simulink model "psbwindgen"  (Simulink 6.0)
settings: Solver=ode23tb  StartTime=0.0  StopTime=3  RelTol=1e-4
PreLoadFcn:
  | load psbwindgen_data
InitFcn:
  | powericon('psbinitsys',bdroot);
values from neighbouring files (symbols this model uses):
  psbwindgen_char = [0 0 0 0 0 0 0 0 0 0 0.02551 0.02551 ... (243 elements, 9x27)]    [power_windgen_init.mat]
undefined symbols (not defined in the file or in its folder): gcbh, powericon
libraries: powerlib2 x50, powerlib_extras x5
(part 1 of 2)
settings Model: Creator=gagnonr  LastModifiedBy=batserve  ExtModeAutoUpdateStatusClock=off  ProdHWDeviceType=Specified
settings DataIOCC: LimitDataPoints=off  LoadInitialState=on  SaveFinalState=on  SaveOutput=off  SignalLoggingName=sigsOut
settings OptimizationCC: BlockReduction=off  BooleanDataType=off
settings DebuggingCC: CheckExecutionContextPreStartOutputMsg=on  CheckExecutionContextRuntimeOutputMsg=on  SolverPrmCheckMsg=none
settings HardwareCC: ProdBitPerShort=32  ProdBitPerInt=16  ProdHWDeviceType=Specified  TargetUnknown=on

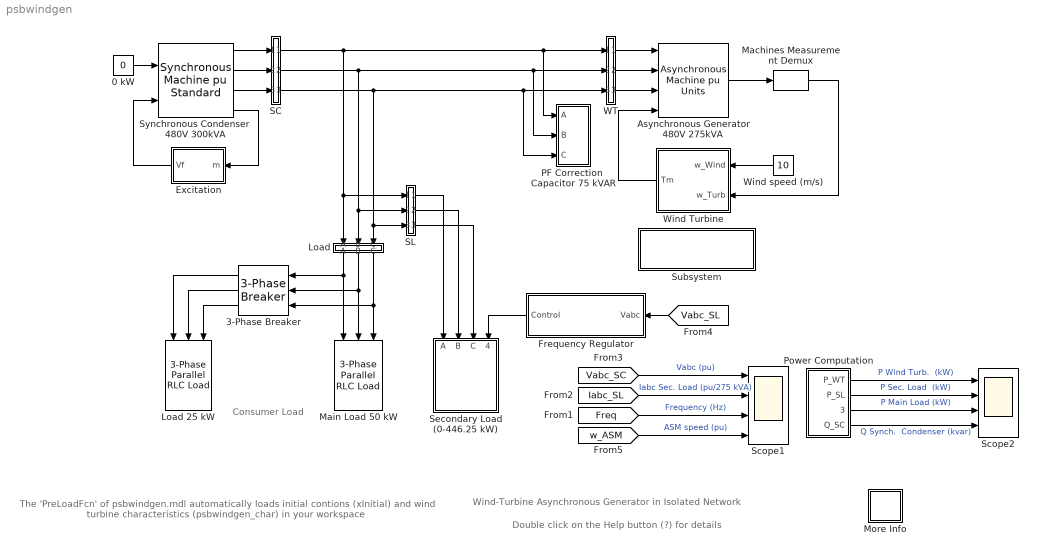
== system psbwindgen ==
  note: Double click on the Help button (?) for details
  note: Wind-Turbine Asynchronous Generator in Isolated Network
  note: The 'PreLoadFcn' of psbwindgen.mdl automatically
      | loads initial contions (xInitial)
      | and wind turbine characteristics (psbwindgen_char)
      | in your workspace
  note: Consumer Load
  0 kW : Constant  Value=0
  3-Phase Breaker : powerlib2/Elements/3-Phase Breaker  Orientation=left  init_states=open  sa=on  sb=on  sc=on  sw_times=[0.2]  Ts=0  comext=off  Ron=0.001  Rp=1e6  Cp=inf  mesure=None
  Asynchronous Generator 480V 275kVA : powerlib2/Machines/Asynchronous Machine pu Units  Tag=PoWeRsYsTeMbLoCk  rotType=Squirrel-cage  ctrl=Rotor  x1=[ 275e3, 480, 60 ]  x2=[ 0.016,0.06]  x3=[ 0.015,0.06]  x4=3.5  x5=[ 2,0,2 ]  x6=[-8.89496e-048 0 0.280896 0.280896 0.280896 -89.7425 150.258 30.2575]  PSBOutputType=1110  iounits=0  LoadFlowParameters=0
  Excitation : Subsystem  Orientation=left
  Frequency Regulator : Subsystem  Orientation=left  mask(Frequency regulator){Vpp_nom=460, Freq=60, gains_regulator=[150 70], Phref=1}
      mask prompts: Vpp_nom "Phase to phase voltage (Vrms):"; Freq "Reference frequency (Hz):"; gains_regulator "Regulator gains  [Kp Kd]:"; Phref "Reference phase (rd):"
      mask help:
      | Frequency regulator
      |
      | Input : phase to ground voltages
      |
      | Output : 24 logical signals for the control of the dump load
      mask init:
      | Vbase=Vpp_nom/sqrt(3);
      | Kp=gains_regulator(1);
      | Kd=gains_regulator(2);
  Load : Subsystem  Tag=PoWeRsYsTeMmEaSuReMeNt  Orientation=down  AncestorBlock=powerlib2/Measurements/Three-Phase V-I Measurement  LoadFcn=powericon('psbloadfunction',gcbh,'3-Phase VI Measurement','');  InitFcn=powericon('checksum',bdroot)  mask(3-Phase VI Measurement){VChoice=phase-to-ground, ualv=on, labelV=Vabc_Load, Vpu=on, Vbase=480, IChoice=yes, ualc=on, labelC=Iabc_Load, Ppu=on, Pbase=275e3, OutputType=Magnitude, PhasorSimulation=off, PSBequivalent=0, PSBOutputType=11100}
      mask prompts: VChoice "Voltage measurement"; ualv "Use a label"; labelV "Signal label  (use a From block to collect signal)"; Vpu "Voltage  in pu"; Vbase "Base voltage (Vrms phase-phase) :"; IChoice "Current measurement"; ualc "Use a label"; labelC "Signal label  (use a From block to collect signal)"; Ppu "Currents in pu"; Pbase "Base power ( VA 3 phase)"; OutputType "Output signal :"; PhasorSimulation "Phasor simulation"; PSBequivalent "Equivalent circuit"
      mask help:
      | This block is used to measure three-phase voltages and currents in a circuit. When connected in series with a three-phase element, it return the three phase-to-ground voltages and line currents.
      |
      | The block can output the voltages and currents in per unit values or in volts and amperes. Check the appropriate boxes if you want to output the voltages and currents  in pu
      mask init:
      | powericon('psbcallbacks',gcb,'Three-phase measurements',4);
      | if  Vpu
      |     xKv=1/(Vbase/sqrt(3)*sqrt(2));
      | else
      |     xKv=1;
      | end
      | if  Ppu
      |     xKi=1/(Pbase/Vbase/sqrt(3)*sqrt(2));
      | else
      |     xKi=1;
      | end
      | switch OutputType
      | case 1
      |     OutputSelection  = [1:6];
      |     PhasorModeV = [1:3];
      |     NormalModeV = [7:9];
      |     PhasorModeI = [4:6];
      |     NormalModeI = [10:12];
      |     Kv = xKv;
      |     Ki = xKi;
      | case 2
      |     OutputSelection = [7,13,8,14,9,15,10,16,11,17,12,18];
      |     PhasorModeV = [1:6];
      |     NormalModeV = [13:15];
      |     PhasorModeI = [7:12];
      |     NormalModeI = [16:18];
      |     Kv = xKv;
      |     Ki = xKi;
      | case 3
      |     OutputSelection = [13,19,14,20,15,21,16,22,17,23,18,24];
      |     PhasorModeV = [1:6];
      |     NormalModeV = [13:15];
      |     PhasorModeI = [7:12];
      |     NormalModeI = [16:18];
      |     Kv = [xKv 1 xKv 1 xKv 1];
      |     Ki = [xKi 1 xKi 1 xKi 1];
      | case 4
      |     OutputSelection  = [19:24];
      |     PhasorModeV = [1:3];
      |     NormalModeV = [7:9];
      |     PhasorModeI = [4:6];
      |     NormalModeI = [10:12];
      |     Kv = xKv;
      |     Ki = xKi;
      | end
      | if PhasorSimulation
      |     SelectionModeV = PhasorModeV;
      |     SelectionModeI = PhasorModeI;
      | else
      |     SelectionModeV = NormalModeV;
      |     SelectionModeI = NormalModeI;
      |     Kv = xKv;
      |     Ki = xKi;
      | end
      settings: CopyFcn=powericon('psbloadfunction',gcbh,'3-Phase VI Measurement','VerifyPhasor');  CloseFcn=%3phaseVImeasurement
      mask Help: web(psbhelp)
      mask StyleString: popup(no|phase-to-ground|phase-to-phase),checkbox,edit,checkbox,edit,popup(no|yes),checkbox,edit,checkbox,edit,popup(Complex|Real-Imag|Magnitude-Angle|Magnitude),checkbox,edit,edit
      mask CallbackString: powericon('psbcallbacks',gcb,'Three-phase measurements',2);|powericon('psbcallbacks',gcb,'Three-phase measurements',2);||powericon('psbcallbacks',gcb,'Three-phase measurements',2);||powericon('psbcallbacks',gcb,'Three-phase measurements',2);|powericon('psbcallbacks',gcb,'Three-phase measurements',2);||powericon('psbcallbacks',gcb,'Three-phase measurements',4);|||||
  Load 25 kW : powerlib2/Elements/3-Phase Parallel RLC Load  Orientation=down  Vpp=480  fn=60  P3=25e3  QL3=0  QC3=0
  Machines Measurement Demux : powerlib2/Machines/Machines Measurement Demux  machType=Asynchronous  ssm1=on  ssm2=on  ssm3=on  ssm4=on  ssm5=on  ssm6=on  sm1=off  sm2=off  sm3=off  sm4=off  sm5=off  sm6=off  sm7=off  sm8=on  sm9=off  sm10=off  sm11=off  sm115=off  sm12=off  sm13=off  sm14=off  asm1=off  asm2=off  asm3=off  asm4=off  asm5=off  asm6=off  asm7=off  asm8=off  asm9=on  asm10=off  asm11=off  pmsm1=on  pmsm2=on  pmsm3=on  pmsm4=on  pmsm5=on  pmsm6=on  lastType=1
  Main Load 50 kW : powerlib2/Elements/3-Phase Parallel RLC Load  Orientation=down  Vpp=480  fn=60  P3=50e3  QL3=0  QC3=0
  More Info : Subsystem
      mask Display: disp('?')
  PF Correction  Capacitor 75 kVAR : Subsystem
  Power Computation : Subsystem
  SC : Subsystem  Tag=PoWeRsYsTeMmEaSuReMeNt  AncestorBlock=powerlib2/Measurements/Three-Phase V-I Measurement  LoadFcn=powericon('psbloadfunction',gcbh,'3-Phase VI Measurement','');  InitFcn=powericon('checksum',bdroot)  mask(3-Phase VI Measurement){VChoice=phase-to-ground, ualv=on, labelV=Vabc_SC, Vpu=on, Vbase=480, IChoice=yes, ualc=on, labelC=Iabc_SC, Ppu=on, Pbase=300e3, OutputType=Magnitude, PhasorSimulation=off, PSBequivalent=0, PSBOutputType=11100}
      mask prompts: VChoice "Voltage measurement"; ualv "Use a label"; labelV "Signal label  (use a From block to collect signal)"; Vpu "Voltage  in pu"; Vbase "Base voltage (Vrms phase-phase) :"; IChoice "Current measurement"; ualc "Use a label"; labelC "Signal label  (use a From block to collect signal)"; Ppu "Currents in pu"; Pbase "Base power ( VA 3 phase)"; OutputType "Output signal :"; PhasorSimulation "Phasor simulation"; PSBequivalent "Equivalent circuit"
      mask help:
      | This block is used to measure three-phase voltages and currents in a circuit. When connected in series with a three-phase element, it return the three phase-to-ground voltages and line currents.
      |
      | The block can output the voltages and currents in per unit values or in volts and amperes. Check the appropriate boxes if you want to output the voltages and currents  in pu
      mask init: same as psbwindgen/Load
      settings: CopyFcn=powericon('psbloadfunction',gcbh,'3-Phase VI Measurement','VerifyPhasor');  CloseFcn=%3phaseVImeasurement
      mask Help: web(psbhelp)
      mask StyleString: popup(no|phase-to-ground|phase-to-phase),checkbox,edit,checkbox,edit,popup(no|yes),checkbox,edit,checkbox,edit,popup(Complex|Real-Imag|Magnitude-Angle|Magnitude),checkbox,edit,edit
      mask CallbackString: powericon('psbcallbacks',gcb,'Three-phase measurements',2);|powericon('psbcallbacks',gcb,'Three-phase measurements',2);||powericon('psbcallbacks',gcb,'Three-phase measurements',2);||powericon('psbcallbacks',gcb,'Three-phase measurements',2);|powericon('psbcallbacks',gcb,'Three-phase measurements',2);||powericon('psbcallbacks',gcb,'Three-phase measurements',4);|||||
  SL : Subsystem  Tag=PoWeRsYsTeMmEaSuReMeNt  AncestorBlock=powerlib2/Measurements/Three-Phase V-I Measurement  LoadFcn=powericon('psbloadfunction',gcbh,'3-Phase VI Measurement','');  InitFcn=powericon('checksum',bdroot)  mask(3-Phase VI Measurement){VChoice=phase-to-ground, ualv=on, labelV=Vabc_SL, Vpu=on, Vbase=480, IChoice=yes, ualc=on, labelC=Iabc_SL, Ppu=on, Pbase=275e3, OutputType=Magnitude, PhasorSimulation=off, PSBequivalent=0, PSBOutputType=11100}
      mask prompts: VChoice "Voltage measurement"; ualv "Use a label"; labelV "Signal label  (use a From block to collect signal)"; Vpu "Voltage  in pu"; Vbase "Base voltage (Vrms phase-phase) :"; IChoice "Current measurement"; ualc "Use a label"; labelC "Signal label  (use a From block to collect signal)"; Ppu "Currents in pu"; Pbase "Base power ( VA 3 phase)"; OutputType "Output signal :"; PhasorSimulation "Phasor simulation"; PSBequivalent "Equivalent circuit"
      mask help:
      | This block is used to measure three-phase voltages and currents in a circuit. When connected in series with a three-phase element, it return the three phase-to-ground voltages and line currents.
      |
      | The block can output the voltages and currents in per unit values or in volts and amperes. Check the appropriate boxes if you want to output the voltages and currents  in pu
      mask init: same as psbwindgen/Load
      settings: CopyFcn=powericon('psbloadfunction',gcbh,'3-Phase VI Measurement','VerifyPhasor');  CloseFcn=%3phaseVImeasurement
      mask Help: web(psbhelp)
      mask StyleString: popup(no|phase-to-ground|phase-to-phase),checkbox,edit,checkbox,edit,popup(no|yes),checkbox,edit,checkbox,edit,popup(Complex|Real-Imag|Magnitude-Angle|Magnitude),checkbox,edit,edit
      mask CallbackString: powericon('psbcallbacks',gcb,'Three-phase measurements',2);|powericon('psbcallbacks',gcb,'Three-phase measurements',2);||powericon('psbcallbacks',gcb,'Three-phase measurements',2);||powericon('psbcallbacks',gcb,'Three-phase measurements',2);|powericon('psbcallbacks',gcb,'Three-phase measurements',2);||powericon('psbcallbacks',gcb,'Three-phase measurements',4);|||||
  Scope1 : Scope  NumInputPorts=4
      settings: TimeRange=3  YMin=-1.5~-0.75~59.5~1.005  YMax=1.5~0.75~60.5~1.015  SaveName=Vabc
  Scope2 : Scope  NumInputPorts=4
      settings: TimeRange=3  YMin=180~100~40~0  YMax=250~200~80~35  SaveName=Power  DataFormat=Array
  Secondary Load (0-446.25 kW) : Subsystem  Orientation=down  mask(8-step Variable Load){Vphase_phase_lissage=480, Freq=60, P_lissage_min=1.75e3, Pin_3phase=50e3}
      mask prompts: Vphase_phase_lissage "Nominal L-L voltage (Vrms):"; Freq "Nominal frequency (Hz):"; P_lissage_min "Power per step Pstep (W):"; Pin_3phase "Initial power  (W) :"
      mask help:
      | This block implements a variable, three-phase resistive load. The load variation uses an eight-bit binary progression so that the load power can be varied by steps from 0 to 255*Pstep.
      |
      | The eight three-phase resistors are connected in series with ideal switches simulating forced-commutated power electronic switches.
      |
      | The Pulses input is a vector containing the eight bits (0/1) controlling the eight three-phase switches. First value is the less significant bit.
      mask init:
      | Ron_switch=1e-6;
      | Rs_snubber=inf;
      | Cs_snubber=0;
      | n_niveaux=8;
      | Pmax=((2^n_niveaux)-1)*P_lissage_min;
      | Pin_normalise=min([(Pin_3phase/Pmax)*((2^n_niveaux)-1) ((2^n_niveaux)-1)]);
      | discret1=pow2(0:-1:-(n_niveaux-1))*Pin_normalise;
      | discret2=floor(discret1);
      | Status=rem(discret2,2);
  Subsystem : Subsystem
      settings: OpenFcn=open('psbwindgen_turb.fig')
      mask Display: disp('Double click to display\nTurbine characteristics')
  Synchronous Condenser  480V 300kVA : powerlib2/Machines/Synchronous Machine pu Standard  Tag=PoWeRsYsTeMbLoCk  rotorType=Salient-pole  x1=[ 300e3 480 60 ]  x2b=[ 3.23, 0.21, 0.15, 2.79, 1.03, 0.37, 0.09 ]  x2=[ 3.23, 0.21, 0.15, 2.79, 0.37, 0.09]  dAxisT=Open-circuit  qAxisT=Open-circuit  x3a="[ 1.7  0.008  0.004]"  x3b=[ 1.7, 0.008, 0.213, 0.004 ]  x3c="[  1.7 0.008 0.051266  ]"  x3d=[ 8.0, 0.03, 0.3371, 0.0295 ]  x3="[ 0.08  0.019  0.004 ]"  x3e=[ 1.3201, 0.023, 1.0, 0.07 ]  x3f="[  0.08  0.019 0.051266  ]"  x3g=[ 1.3201, 0.0231, 0.3371, 0.0295 ]  x4=0.017  x5=[ 1, 0, 2 ]  x6=[0 -89.2146 0.827 0.827 0.827 -86.4 153.6 33.6 2.71455]  x7=off  x8=[0.6404,0.7127,0.8441,0.9214,0.9956,1.082,1.19,1.316,1.457;0.7,0.7698,0.8872,0.9466,0.9969,1.046,1.1,1.151,1.201]  PSBOutputType=1110  iounits=0.5  LoadFlowParameters=[2 0 0 0 0]
  WT : Subsystem  Tag=PoWeRsYsTeMmEaSuReMeNt  AncestorBlock=powerlib2/Measurements/Three-Phase V-I Measurement  LoadFcn=powericon('psbloadfunction',gcbh,'3-Phase VI Measurement','');  InitFcn=powericon('checksum',bdroot)  mask(3-Phase VI Measurement){VChoice=phase-to-ground, ualv=on, labelV=Vabc_WT, Vpu=on, Vbase=480, IChoice=yes, ualc=on, labelC=Iabc_WT, Ppu=on, Pbase=275e3, OutputType=Magnitude, PhasorSimulation=off, PSBequivalent=0, PSBOutputType=11100}
      mask prompts: VChoice "Voltage measurement"; ualv "Use a label"; labelV "Signal label  (use a From block to collect signal)"; Vpu "Voltage  in pu"; Vbase "Base voltage (Vrms phase-phase) :"; IChoice "Current measurement"; ualc "Use a label"; labelC "Signal label  (use a From block to collect signal)"; Ppu "Currents in pu"; Pbase "Base power ( VA 3 phase)"; OutputType "Output signal :"; PhasorSimulation "Phasor simulation"; PSBequivalent "Equivalent circuit"
      mask help:
      | This block is used to measure three-phase voltages and currents in a circuit. When connected in series with a three-phase element, it return the three phase-to-ground voltages and line currents.
      |
      | The block can output the voltages and currents in per unit values or in volts and amperes. Check the appropriate boxes if you want to output the voltages and currents  in pu
      mask init: same as psbwindgen/Load
      settings: CopyFcn=powericon('psbloadfunction',gcbh,'3-Phase VI Measurement','VerifyPhasor');  CloseFcn=%3phaseVImeasurement
      mask Help: web(psbhelp)
      mask StyleString: popup(no|phase-to-ground|phase-to-phase),checkbox,edit,checkbox,edit,popup(no|yes),checkbox,edit,checkbox,edit,popup(Complex|Real-Imag|Magnitude-Angle|Magnitude),checkbox,edit,edit
      mask CallbackString: powericon('psbcallbacks',gcb,'Three-phase measurements',2);|powericon('psbcallbacks',gcb,'Three-phase measurements',2);||powericon('psbcallbacks',gcb,'Three-phase measurements',2);||powericon('psbcallbacks',gcb,'Three-phase measurements',2);|powericon('psbcallbacks',gcb,'Three-phase measurements',2);||powericon('psbcallbacks',gcb,'Three-phase measurements',4);|||||
  Wind Turbine : Subsystem  Orientation=left
  Wind speed (m/s) : Constant  Orientation=left  Value=10
  wires:
  Load/3("C ") -> Main Load 50 kW/3, 3-Phase Breaker/3
  0 kW/1 -> Synchronous Condenser  480V 300kVA/1
  Synchronous Condenser  480V 300kVA/4 -> Excitation/1(m)
  Excitation/1(Vf) -> Synchronous Condenser  480V 300kVA/2
  [Freq] -> Scope1/3  "Frequency (Hz)"
  [Vabc_SC] -> Scope1/1  "Vabc (pu)"
  Load/1("A ") -> Main Load 50 kW/1, 3-Phase Breaker/1
  Load/2("B ") -> Main Load 50 kW/2, 3-Phase Breaker/2
  WT/1("A ") -> Asynchronous Generator 480V 275kVA/1
  WT/2("B ") -> Asynchronous Generator 480V 275kVA/2
  WT/3("C ") -> Asynchronous Generator 480V 275kVA/3
  Synchronous Condenser  480V 300kVA/1 -> SC/1(A)
  Synchronous Condenser  480V 300kVA/2 -> SC/2(B)
  Synchronous Condenser  480V 300kVA/3 -> SC/3(C)
  SC/1("A ") -> PF Correction  Capacitor 75 kVAR/1(A), WT/1(A), SL/1(A), Load/1(A)
  SC/2("B ") -> PF Correction  Capacitor 75 kVAR/2(B), WT/2(B), SL/2(B), Load/2(B)
  SC/3("C ") -> PF Correction  Capacitor 75 kVAR/3(C), WT/3(C), SL/3(C), Load/3(C)
  [Iabc_SL] -> Scope1/2  "Iabc Sec. Load (pu/275 kVA)"
  3-Phase Breaker/1 -> Load 25 kW/1
  3-Phase Breaker/2 -> Load 25 kW/2
  3-Phase Breaker/3 -> Load 25 kW/3
  Asynchronous Generator 480V 275kVA/1 -> Machines Measurement Demux/1
  Machines Measurement Demux/1 -> Wind Turbine/2(w_Turb)
  Wind speed (m/s)/1 -> Wind Turbine/1(w_Wind)
  [Vabc_SL] -> Frequency Regulator/1(Vabc)
  Power Computation/1(P_WT) -> Scope2/1  "P Wind Turb.  (kW)"
  Power Computation/2(P_SL) -> Scope2/2  "P Sec. Load  (kW)"
  Power Computation/3(P_Load) -> Scope2/3  "P Main Load (kW)"
  Power Computation/4(Q_SC) -> Scope2/4  "Q Synch.  Condenser (kvar)"
  Wind Turbine/1(Tm) -> Asynchronous Generator 480V 275kVA/4
  SL/1("A ") -> Secondary Load (0-446.25 kW)/1(A)
  SL/2("B ") -> Secondary Load (0-446.25 kW)/2(B)
  SL/3("C ") -> Secondary Load (0-446.25 kW)/3(C)
  Frequency Regulator/1(Control) -> Secondary Load (0-446.25 kW)/4(Control)
  [w_ASM] -> Scope1/4  "ASM speed (pu)"

== system psbwindgen/Excitation ==
  m : Inport  Orientation=left  Port=1  LatchInput=off
  Constant3 : Constant  Orientation=left
  Demux : Demux  Orientation=left  Outputs=2
  Excitation System : powerlib2/Machines/Excitation System  Orientation=left  tr=20e-3  reg=[ 300, 0.001 ]  exc=[ 1, 0 ]  tgr=[ 0, 0 ]  damp=[ 0.001, 0.1 ]  sat=[ 0, 0 ]  lim=[ -11.5, 11.5, 0 ]  v0=[1,2.71455]
  Gain : Gain  Gain=60  SaturateOnIntegerOverflow=on
  Ground : Ground  Orientation=left
  Machines Measurement Demux : powerlib2/Machines/Machines Measurement Demux  Orientation=left  machType=Synchronous  ssm1=on  ssm2=on  ssm3=on  ssm4=on  ssm5=on  ssm6=on  sm1=off  sm2=off  sm3=off  sm4=off  sm5=off  sm6=on  sm7=off  sm8=on  sm9=off  sm10=off  sm11=off  sm115=off  sm12=off  sm13=off  sm14=off  asm1=on  asm2=on  asm3=on  asm4=on  asm5=on  asm6=on  asm7=on  asm8=on  asm9=on  asm10=on  asm11=on  pmsm1=on  pmsm2=on  pmsm3=on  pmsm4=on  pmsm5=on  pmsm6=on  lastType=1
  Vf : Outport  Orientation=left
  tag scope: Freq=global
  wires:
  Machines Measurement Demux/1 -> Demux/1
  Demux/1 -> Excitation System/3
  Demux/2 -> Excitation System/2
  Constant3/1 -> Excitation System/1
  Ground/1 -> Excitation System/4
  Machines Measurement Demux/2 -> Gain/1
  m/1 -> Machines Measurement Demux/1
  Excitation System/1 -> Vf/1
  Gain/1 -> [Freq]

== system psbwindgen/Frequency Regulator ==
  Vabc : Inport  Port=1  LatchInput=off
  3-phase PLL : powerlib_extras/Control  Blocks/3-phase PLL  Par_Init=[0 Freq]  ParK=[60 1400]
  Frequency : Constant  Value=Freq
  Integrator : Integrator  LimitOutput=on  UpperSaturationLimit=6  LowerSaturationLimit=-1
  PD : Subsystem
  Phref : Constant  Value=Phref
  Pulses Decoder : Subsystem  mask(Pulses Decoder){n=8}
      mask prompts: n "Number of bits to decode:"
      mask help:
      | Decode the scalar input 'Code' into a vector output 'Pulses' based on  the specified number of bits to decode.
      | (Element 1 of vector output = least significant bit)
  Sampling system : Subsystem
  Sum : Sum  Inputs=|+-  SaturateOnIntegerOverflow=on  InputSameDT=on
  Sum1 : Sum  Inputs=|+-  SaturateOnIntegerOverflow=on  InputSameDT=on
  Terminator : Terminator
  Terminator1 : Terminator
  Control : Outport
  wires:
  Vabc/1 -> 3-phase PLL/1
  3-phase PLL/3 -> Terminator1/1
  3-phase PLL/2 -> Terminator/1
  3-phase PLL/1 -> Sum/1
  Sampling system/1(Pulses_ABC0_7) -> Control/1
  Phref/1 -> Sum1/2
  Sum1/1 -> PD/1(In)
  Integrator/1 -> Sum1/1
  Frequency/1 -> Sum/2
  PD/1(Out) -> Pulses Decoder/1(Code)
  Sum/1 -> Integrator/1
  Pulses Decoder/1(Pulses) -> Sampling system/1(BITA0_7)

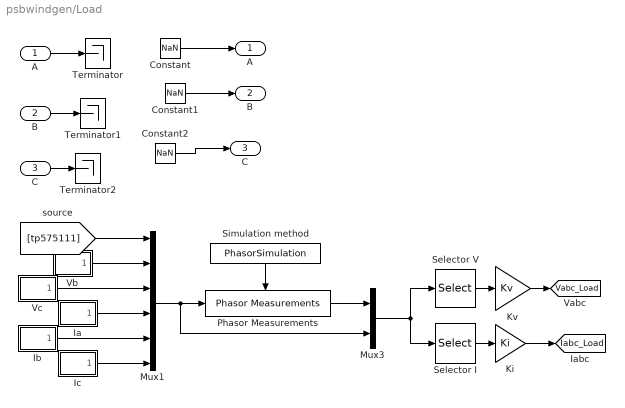
== system psbwindgen/Load ==
  A : Inport  Port=1  LatchInput=off
  B : Inport  Port=2  LatchInput=off
  C : Inport  Port=3  LatchInput=off
  Constant : Constant  Value=NaN
  Constant1 : Constant  Value=NaN
  Constant2 : Constant  Value=NaN
  Ia : Subsystem  AncestorBlock=powerlib2/Measurements/Three-Phase V-I Measurement/Ia
  Ib : Subsystem  AncestorBlock=powerlib2/Measurements/Three-Phase V-I Measurement/Ib
  Ic : Subsystem  AncestorBlock=powerlib2/Measurements/Three-Phase V-I Measurement/Ic
  Ki : Gain  Gain=Ki  SaturateOnIntegerOverflow=on
  Kv : Gain  Gain=Kv  SaturateOnIntegerOverflow=on
  Mux1 : Mux  Inputs=6
  Mux3 : Mux  Inputs=2
  Phasor Measurements : powerlib2/Measurements/Three-Phase V-I Measurement/Phasor Measurements  TreatAsAtomicUnit=on  SimViewingDevice=off  DataTypeOverride=UseLocalSettings  MinMaxOverflowLogging=UseLocalSettings
      settings: Permissions=ReadWrite  RTWFcnNameOpts=Auto  RTWFileNameOpts=Auto
  Selector I : Selector  Elements=SelectionModeI  InputPortWidth=length(OutputSelection)+6
  Selector V : Selector  Elements=SelectionModeV  InputPortWidth=length(OutputSelection)+6
  Simulation method : Constant  Orientation=down  Value=PhasorSimulation
  Terminator : Terminator
  Terminator1 : Terminator
  Terminator2 : Terminator
  Vb : Subsystem  AncestorBlock=powerlib2/Measurements/Three-Phase V-I Measurement/Vb
  Vc : Subsystem  AncestorBlock=powerlib2/Measurements/Three-Phase V-I Measurement/Vc
  "A " : Outport
  "B " : Outport  Port=2
  "C " : Outport  Port=3
  tag scope: Iabc_Load=global, Vabc_Load=global
  wires:
  Ic/1(Out1) -> Mux1/6
  Ib/1(Out1) -> Mux1/5
  Ia/1(Out1) -> Mux1/4
  Vc/1(Out1) -> Mux1/3
  Vb/1(Out1) -> Mux1/2
  [tp575111] -> Mux1/1
  Mux1/1 -> Phasor Measurements/1, Mux3/2
  Simulation method/1 -> Phasor Measurements/Enable
  Phasor Measurements/1 -> Mux3/1
  Mux3/1 -> Selector V/1, Selector I/1
  Selector I/1 -> Ki/1
  Selector V/1 -> Kv/1
  Ki/1 -> [Iabc_Load]
  Kv/1 -> [Vabc_Load]
  Constant2/1 -> "C "/1
  Constant1/1 -> "B "/1
  Constant/1 -> "A "/1
  C/1 -> Terminator2/1
  B/1 -> Terminator1/1
  A/1 -> Terminator/1

== system psbwindgen/More Info ==
  note: [1] R. Gagnon, B. Saulnier, G. Sybille, P. Giroux; "Modeling of a Generic High-Penetration No-Storage Wind-Diesel System Using Matlab/Power System Blockset"
      | 2002 Global Windpower Conference, April 2002, Paris, France
      | [2] B. Saulnier, A.O. Barry, B. Dube, R. Reid; "Design and Development of a Regulation and Control System for the High-Penetration No-Storage Wind/Diesel
      | Scheme" European Community Wind Energy Conference 88, 6-10 june 1988, Herning, Denmark
      | [3] L. Mott (NPS), B. Saulnier (IREQ) " Commercial Wind-Diesel Project, St. Paul Island, Alaska" 14th Prime Power Diesel Inter-Utility Conference,
      | May 28-June 2, Winnipeg, Manitoba, Canada
  note: References
  note: For the demo, the wind speed (10m/s) is such that the wind turbine produces enough power to supply the load. The diesel-generator (not simulated) is stopped
      | and the the synchronous machine operates as a synchronous condenser with its mechanical power input (Pm) set at zero.
      | The demo illustrates the dynamic performance of the frequency regulation system when an additional 25 kW customer load is switched on.
      |
      | Start simulation and observe voltages, currents, powers, asynchronous machine speed and system frequency on the two scopes.
      | Initial conditions (xInitial vector) have been automatically loaded in your workspace so that simulation starts in steady state.
      |
      | As the asynchronous machine operates in generator mode, its speed is slightly above the synchronous speed (1.011 pu).
      | According to turbine characteristics, for a 10m/s wind speed, the turbine output power is 0.75 pu (206 kW). Because of the asynchronous machine losses,
      | the wind turbine produces 200 kW. As the main load is 50 kW, the secondary load absorbs 150 kW to maintain a constant 60 Hz frequency.
      | At t=0.2 s, the additional load of 25 kW is switched on. The frequency  momentarily drops to 59.8 Hz and the frequency regulator reacts to reduce the power
      | absorbed by the secondary load in order to bring the frequency back to 60 Hz. Voltage stays at 1 pu and no flicker is observed.
  note: R. Reid, B. Saulnier, R. Gagnon; Hydro-Quebec (IREQ)
  note: A generic model of the High-Penetration, No Storage, Wind-Diesel (HPNSWD) system is presented in this demo [1].
      | This technology was developed by Hydro-Quebec to reduce the cost of supplying electricity in remote northern communities[2].
      | The optimal wind penetration (installed wind capacity/peak electrical demand) for this system depends on the site delivery cost of fuel
      | and available wind resource. The first commercial application of HPNSWD technology was commissioned in 1999 by Northern Power Systems (Vermont,USA)
      | on St. Paul Island, Alaska [3]. The HPNSWD system presented in this demo uses a 480 V, 300 kVA synchronous machine, a wind turbine driving
      | a 480 V, 275 kVA induction generator, a 50 kW customer load and a variable secondary load (0 to 446.25 kW).
      |
      | At low wind speeds both the induction generator and the diesel-driven synchronous generator are required to feed the load.
      | When the wind power exceeds the load demand, it is possible to shut down the diesel-generator. In this all-wind mode, the synchronous machine
      | is used as a synchronous condenser and its excitation system controls the grid voltage at its nominal value.
      | A secondary load bank is used to regulate the system frequency by absorbing the wind power exceeding consumer demand.
      |
      | The Wind Turbine block uses a 2-D Lookup Table to compute the turbine torque output (Tm) as a function of wind speed (w_Wind) and turbine speed (w_Turb).
      | When you opened this demo, the Pm(w_Wind, w_Turb) characteristics was automatically loaded in your workspace (psbwindgen_char array).
      | To display the turbine characteristics, double click on the block located below the Wind Turbine block.
      |
      | The Secondary Load block consists of eight sets of three-phase resistors connected in series with GTO thyristor switches.
      | The nominal power of each set follows a binary progression so that the load can be varied from 0 to 446.25 kW by steps of 1.75kW.
      | GTOs are simulated by ideal switches.
      |
      | The Frequency Regulator uses a standard three-phase Phase Locked Loop (PLL) system to measure the system frequency.
      | The measured frequency is compared to the reference frequency (60 Hz) to obtain the frequency error. This error is integrated to obtain the
      | phase error. The phase error is then used  by a Proportional-Differential (PD) controller to produce an output signal representing the required
      | secondary load power. This analog signal is converted to an 8-bit digital signal controlling switching of the eight three-phase secondary loads.
      | In order to minimize voltage disturbances, switching is performed at zero crossing of voltage.
  note: Wind-Turbine Asynchronous Generator in Isolated Network
  note: Circuit Description
  note: Demonstration

== system psbwindgen/PF Correction  Capacitor 75 kVAR ==
  A : Inport  Orientation=left  Port=1  LatchInput=off
  B : Inport  Orientation=left  Port=2  LatchInput=off
  C : Inport  Orientation=left  Port=3  LatchInput=off
  L connector : powerlib2/Connectors/L connector  Tag=PoWeRsYsTeMbLoCk
  L connector1 : powerlib2/Connectors/L connector  Tag=PoWeRsYsTeMbLoCk
  L connector2 : powerlib2/Connectors/L connector  Tag=PoWeRsYsTeMbLoCk
  Series RLC Load : powerlib2/Elements/Series RLC Load  Tag=PoWeRsYsTeMbLoCk  a=480  b=60  c=0  d=0  e=25e3  mesure=None  PSBOutputType=1
  Series RLC Load2 : powerlib2/Elements/Series RLC Load  Tag=PoWeRsYsTeMbLoCk  a=480  b=60  c=0  d=0  e=25e3  mesure=None  PSBOutputType=1
  Series RLC Load3 : powerlib2/Elements/Series RLC Load  Tag=PoWeRsYsTeMbLoCk  a=480  b=60  c=0  d=0  e=25e3  mesure=None  PSBOutputType=1
  wires:
  C/1 -> L connector2/Enable
  B/1 -> L connector1/Enable
  A/1 -> L connector/Enable
  Series RLC Load2/1 -> L connector2/1, Series RLC Load/1
  Series RLC Load3/1 -> L connector1/1, Series RLC Load2/1
  Series RLC Load/1 -> L connector/1, Series RLC Load3/1

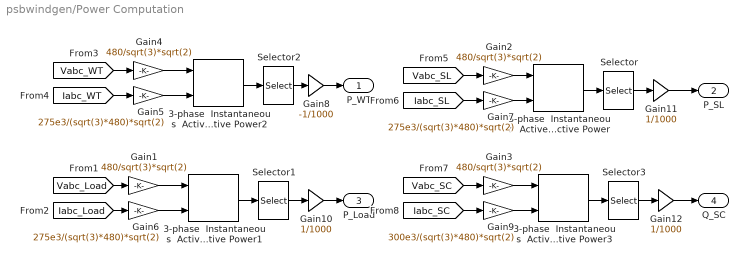
== system psbwindgen/Power Computation ==
  3-phase  Instantaneous  Active & Reactive Power{,1..3} (4 alike) : powerlib_extras/Measurements/3-phase  Instantaneous  Active & Reactive Power
  Gain{1..4} (4 alike) : Gain  Gain=480/sqrt(3)*sqrt(2)  SaturateOnIntegerOverflow=on
  Gain10 : Gain  Gain=1/1000  SaturateOnIntegerOverflow=on
  Gain11 : Gain  Gain=1/1000  SaturateOnIntegerOverflow=on
  Gain12 : Gain  Gain=1/1000  SaturateOnIntegerOverflow=on
  Gain5 : Gain  Gain=275e3/(sqrt(3)*480)*sqrt(2)  SaturateOnIntegerOverflow=on
  Gain6 : Gain  Gain=275e3/(sqrt(3)*480)*sqrt(2)  SaturateOnIntegerOverflow=on
  Gain7 : Gain  Gain=275e3/(sqrt(3)*480)*sqrt(2)  SaturateOnIntegerOverflow=on
  Gain8 : Gain  Gain=-1/1000  SaturateOnIntegerOverflow=on
  Gain9 : Gain  Gain=300e3/(sqrt(3)*480)*sqrt(2)  SaturateOnIntegerOverflow=on
  Selector : Selector  Elements=[1]  InputPortWidth=2
  Selector1 : Selector  Elements=[1]  InputPortWidth=2
  Selector2 : Selector  Elements=[1]  InputPortWidth=2
  Selector3 : Selector  Elements=[2]  InputPortWidth=2
  P_WT : Outport
  P_SL : Outport  Port=2
  P_Load : Outport  Port=3
  Q_SC : Outport  Port=4
  wires:
  3-phase  Instantaneous  Active & Reactive Power/1 -> Selector/1
  Selector/1 -> Gain11/1
  3-phase  Instantaneous  Active & Reactive Power1/1 -> Selector1/1
  3-phase  Instantaneous  Active & Reactive Power2/1 -> Selector2/1
  [Vabc_WT] -> Gain4/1
  [Iabc_WT] -> Gain5/1
  3-phase  Instantaneous  Active & Reactive Power3/1 -> Selector3/1
  Gain4/1 -> 3-phase  Instantaneous  Active & Reactive Power2/1
  Gain5/1 -> 3-phase  Instantaneous  Active & Reactive Power2/2
  [Vabc_Load] -> Gain1/1
  [Iabc_Load] -> Gain6/1
  Gain1/1 -> 3-phase  Instantaneous  Active & Reactive Power1/1
  Gain6/1 -> 3-phase  Instantaneous  Active & Reactive Power1/2
  [Vabc_SL] -> Gain2/1
  [Iabc_SL] -> Gain7/1
  Gain2/1 -> 3-phase  Instantaneous  Active & Reactive Power/1
  Gain7/1 -> 3-phase  Instantaneous  Active & Reactive Power/2
  Selector1/1 -> Gain10/1
  Selector2/1 -> Gain8/1
  Gain8/1 -> P_WT/1
  Selector3/1 -> Gain12/1
  [Vabc_SC] -> Gain3/1
  [Iabc_SC] -> Gain9/1
  Gain3/1 -> 3-phase  Instantaneous  Active & Reactive Power3/1
  Gain9/1 -> 3-phase  Instantaneous  Active & Reactive Power3/2
  Gain10/1 -> P_Load/1
  Gain11/1 -> P_SL/1
  Gain12/1 -> Q_SC/1

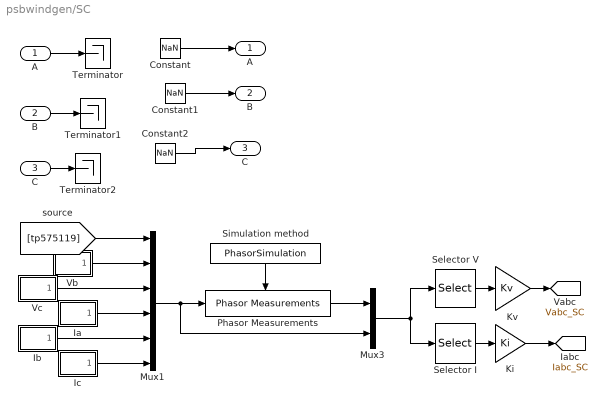
== system psbwindgen/SC ==
  A : Inport  Port=1  LatchInput=off
  B : Inport  Port=2  LatchInput=off
  C : Inport  Port=3  LatchInput=off
  Constant : Constant  Value=NaN
  Constant1 : Constant  Value=NaN
  Constant2 : Constant  Value=NaN
  Ia : Subsystem  AncestorBlock=powerlib2/Measurements/Three-Phase V-I Measurement/Ia
  Ib : Subsystem  AncestorBlock=powerlib2/Measurements/Three-Phase V-I Measurement/Ib
  Ic : Subsystem  AncestorBlock=powerlib2/Measurements/Three-Phase V-I Measurement/Ic
  Ki : Gain  Gain=Ki  SaturateOnIntegerOverflow=on
  Kv : Gain  Gain=Kv  SaturateOnIntegerOverflow=on
  Mux1 : Mux  Inputs=6
  Mux3 : Mux  Inputs=2
  Phasor Measurements : powerlib2/Measurements/Three-Phase V-I Measurement/Phasor Measurements  TreatAsAtomicUnit=on  SimViewingDevice=off  DataTypeOverride=UseLocalSettings  MinMaxOverflowLogging=UseLocalSettings
      settings: Permissions=ReadWrite  RTWFcnNameOpts=Auto  RTWFileNameOpts=Auto
  Selector I : Selector  Elements=SelectionModeI  InputPortWidth=length(OutputSelection)+6
  Selector V : Selector  Elements=SelectionModeV  InputPortWidth=length(OutputSelection)+6
  Simulation method : Constant  Orientation=down  Value=PhasorSimulation
  Terminator : Terminator
  Terminator1 : Terminator
  Terminator2 : Terminator
  Vb : Subsystem  AncestorBlock=powerlib2/Measurements/Three-Phase V-I Measurement/Vb
  Vc : Subsystem  AncestorBlock=powerlib2/Measurements/Three-Phase V-I Measurement/Vc
  "A " : Outport
  "B " : Outport  Port=2
  "C " : Outport  Port=3
  tag scope: Iabc_SC=global, Vabc_SC=global
  wires:
  A/1 -> Terminator/1
  B/1 -> Terminator1/1
  C/1 -> Terminator2/1
  Constant/1 -> "A "/1
  Constant1/1 -> "B "/1
  Constant2/1 -> "C "/1
  Kv/1 -> [Vabc_SC]
  Ki/1 -> [Iabc_SC]
  Selector V/1 -> Kv/1
  Selector I/1 -> Ki/1
  Mux3/1 -> Selector I/1, Selector V/1
  Phasor Measurements/1 -> Mux3/1
  Simulation method/1 -> Phasor Measurements/Enable
  Mux1/1 -> Mux3/2, Phasor Measurements/1
  [tp575119] -> Mux1/1
  Vb/1(Out1) -> Mux1/2
  Vc/1(Out1) -> Mux1/3
  Ia/1(Out1) -> Mux1/4
  Ib/1(Out1) -> Mux1/5
  Ic/1(Out1) -> Mux1/6

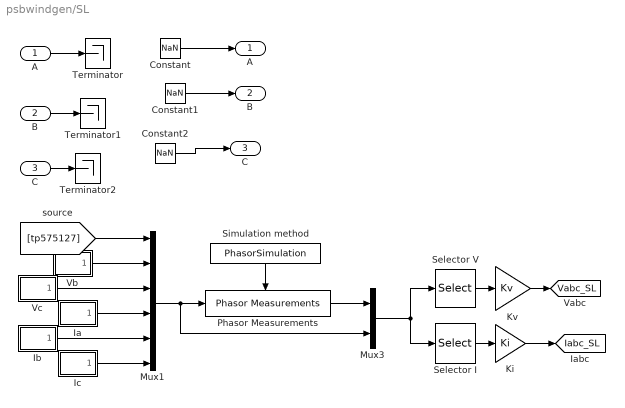
== system psbwindgen/SL ==
  A : Inport  Port=1  LatchInput=off
  B : Inport  Port=2  LatchInput=off
  C : Inport  Port=3  LatchInput=off
  Constant : Constant  Value=NaN
  Constant1 : Constant  Value=NaN
  Constant2 : Constant  Value=NaN
  Ia : Subsystem  AncestorBlock=powerlib2/Measurements/Three-Phase V-I Measurement/Ia
  Ib : Subsystem  AncestorBlock=powerlib2/Measurements/Three-Phase V-I Measurement/Ib
  Ic : Subsystem  AncestorBlock=powerlib2/Measurements/Three-Phase V-I Measurement/Ic
  Ki : Gain  Gain=Ki  SaturateOnIntegerOverflow=on
  Kv : Gain  Gain=Kv  SaturateOnIntegerOverflow=on
  Mux1 : Mux  Inputs=6
  Mux3 : Mux  Inputs=2
  Phasor Measurements : powerlib2/Measurements/Three-Phase V-I Measurement/Phasor Measurements  TreatAsAtomicUnit=on  SimViewingDevice=off  DataTypeOverride=UseLocalSettings  MinMaxOverflowLogging=UseLocalSettings
      settings: Permissions=ReadWrite  RTWFcnNameOpts=Auto  RTWFileNameOpts=Auto
  Selector I : Selector  Elements=SelectionModeI  InputPortWidth=length(OutputSelection)+6
  Selector V : Selector  Elements=SelectionModeV  InputPortWidth=length(OutputSelection)+6
  Simulation method : Constant  Orientation=down  Value=PhasorSimulation
  Terminator : Terminator
  Terminator1 : Terminator
  Terminator2 : Terminator
  Vb : Subsystem  AncestorBlock=powerlib2/Measurements/Three-Phase V-I Measurement/Vb
  Vc : Subsystem  AncestorBlock=powerlib2/Measurements/Three-Phase V-I Measurement/Vc
  "A " : Outport
  "B " : Outport  Port=2
  "C " : Outport  Port=3
  tag scope: Iabc_SL=global, Vabc_SL=global
  wires:
  A/1 -> Terminator/1
  B/1 -> Terminator1/1
  C/1 -> Terminator2/1
  Constant/1 -> "A "/1
  Constant1/1 -> "B "/1
  Constant2/1 -> "C "/1
  Kv/1 -> [Vabc_SL]
  Ki/1 -> [Iabc_SL]
  Selector V/1 -> Kv/1
  Selector I/1 -> Ki/1
  Mux3/1 -> Selector I/1, Selector V/1
  Phasor Measurements/1 -> Mux3/1
  Simulation method/1 -> Phasor Measurements/Enable
  Mux1/1 -> Mux3/2, Phasor Measurements/1
  [tp575127] -> Mux1/1
  Vb/1(Out1) -> Mux1/2
  Vc/1(Out1) -> Mux1/3
  Ia/1(Out1) -> Mux1/4
  Ib/1(Out1) -> Mux1/5
  Ic/1(Out1) -> Mux1/6

== system psbwindgen/Secondary Load (0-446.25 kW) ==
  A : Inport  Port=1  LatchInput=off
  B : Inport  Port=2  LatchInput=off
  C : Inport  Port=3  LatchInput=off
  Control : Inport  Port=4  LatchInput=off
  Demux : Demux  Outputs=8
  Resistive Loads : Subsystem
  Switches : Subsystem
  wires:
  Control/1 -> Demux/1
  Demux/8 -> Switches/11(P_ABC7)
  Demux/7 -> Switches/10(P_ABC6)
  Demux/6 -> Switches/9(P_ABC5)
  Demux/5 -> Switches/8(P_ABC4)
  Demux/4 -> Switches/7(P_ABC3)
  Demux/3 -> Switches/6(P_ABC2)
  Demux/2 -> Switches/5(P_ABC1)
  Demux/1 -> Switches/4(P_ABC0)
  C/1 -> Switches/3(C)
  B/1 -> Switches/2(B)
  A/1 -> Switches/1(A)
  Switches/24(C7) -> Resistive Loads/24(C7)
  Switches/23(B7) -> Resistive Loads/23(B7)
  Switches/22(A7) -> Resistive Loads/22(A7)
  Switches/21(C6) -> Resistive Loads/21(C6)
  Switches/20(B6) -> Resistive Loads/20(B6)
  Switches/19(A6) -> Resistive Loads/19(A6)
  Switches/18(C5) -> Resistive Loads/18(C5)
  Switches/17(B5) -> Resistive Loads/17(B5)
  Switches/16(A5) -> Resistive Loads/16(A5)
  Switches/15(C4) -> Resistive Loads/15(C4)
  Switches/14(B4) -> Resistive Loads/14(B4)
  Switches/13(A4) -> Resistive Loads/13(A4)
  Switches/12(C3) -> Resistive Loads/12(C3)
  Switches/11(B3) -> Resistive Loads/11(B3)
  Switches/10(A3) -> Resistive Loads/10(A3)
  Switches/9(C2) -> Resistive Loads/9(C2)
  Switches/8(B2) -> Resistive Loads/8(B2)
  Switches/7(A2) -> Resistive Loads/7(A2)
  Switches/6(C1) -> Resistive Loads/6(C1)
  Switches/5(B1) -> Resistive Loads/5(B1)
  Switches/4(A1) -> Resistive Loads/4(A1)
  Switches/3(C0) -> Resistive Loads/3(C0)
  Switches/2(B0) -> Resistive Loads/2(B0)
  Switches/1(A0) -> Resistive Loads/1(A0)

== system psbwindgen/Subsystem ==

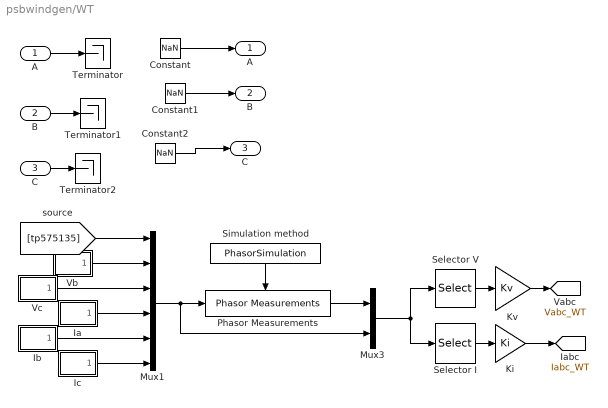
== system psbwindgen/WT ==
  A : Inport  Port=1  LatchInput=off
  B : Inport  Port=2  LatchInput=off
  C : Inport  Port=3  LatchInput=off
  Constant : Constant  Value=NaN
  Constant1 : Constant  Value=NaN
  Constant2 : Constant  Value=NaN
  Ia : Subsystem  AncestorBlock=powerlib2/Measurements/Three-Phase V-I Measurement/Ia
  Ib : Subsystem  AncestorBlock=powerlib2/Measurements/Three-Phase V-I Measurement/Ib
  Ic : Subsystem  AncestorBlock=powerlib2/Measurements/Three-Phase V-I Measurement/Ic
  Ki : Gain  Gain=Ki  SaturateOnIntegerOverflow=on
  Kv : Gain  Gain=Kv  SaturateOnIntegerOverflow=on
  Mux1 : Mux  Inputs=6
  Mux3 : Mux  Inputs=2
  Phasor Measurements : powerlib2/Measurements/Three-Phase V-I Measurement/Phasor Measurements  TreatAsAtomicUnit=on  SimViewingDevice=off  DataTypeOverride=UseLocalSettings  MinMaxOverflowLogging=UseLocalSettings
      settings: Permissions=ReadWrite  RTWFcnNameOpts=Auto  RTWFileNameOpts=Auto
  Selector I : Selector  Elements=SelectionModeI  InputPortWidth=length(OutputSelection)+6
  Selector V : Selector  Elements=SelectionModeV  InputPortWidth=length(OutputSelection)+6
  Simulation method : Constant  Orientation=down  Value=PhasorSimulation
  Terminator : Terminator
  Terminator1 : Terminator
  Terminator2 : Terminator
  Vb : Subsystem  AncestorBlock=powerlib2/Measurements/Three-Phase V-I Measurement/Vb
  Vc : Subsystem  AncestorBlock=powerlib2/Measurements/Three-Phase V-I Measurement/Vc
  "A " : Outport
  "B " : Outport  Port=2
  "C " : Outport  Port=3
  tag scope: Iabc_WT=global, Vabc_WT=global
  wires:
  Ic/1(Out1) -> Mux1/6
  Ib/1(Out1) -> Mux1/5
  Ia/1(Out1) -> Mux1/4
  Vc/1(Out1) -> Mux1/3
  Vb/1(Out1) -> Mux1/2
  [tp575135] -> Mux1/1
  Mux1/1 -> Phasor Measurements/1, Mux3/2
  Simulation method/1 -> Phasor Measurements/Enable
  Phasor Measurements/1 -> Mux3/1
  Mux3/1 -> Selector V/1, Selector I/1
  Selector I/1 -> Ki/1
  Selector V/1 -> Kv/1
  Ki/1 -> [Iabc_WT]
  Kv/1 -> [Vabc_WT]
  Constant2/1 -> "C "/1
  Constant1/1 -> "B "/1
  Constant/1 -> "A "/1
  C/1 -> Terminator2/1
  B/1 -> Terminator1/1
  A/1 -> Terminator/1

== system psbwindgen/Wind Turbine ==
  w_Wind : Inport  Port=1  LatchInput=off
  w_Turb : Inport  Port=2  LatchInput=off
  1800 rpm : Gain  Gain=1800  SaturateOnIntegerOverflow=on
  Constant3 : Constant  Value=1e-6
  Gain : Gain  Gain=-1  SaturateOnIntegerOverflow=on
  P(w_Wind,w_Turb) : Lookup2D  DialogController=Simulink.DDGSource  RowIndex=[0 5 6 7 8 9 10 11 12]  ColumnIndex=[0 571.55 685.8 800.15 914.4 1028.8 1143.1 1257.4 1371.7 1486 1600.3 1714.6 1828.9 1943.2 2057.5 2171.8 2286.1 2400.5 2514.7 2629.1 2743.3 2857.7 2971.9 3086.3 3200.5 3314.9 3429.2]  OutputValues=psbwindgen_char  SaturateOnIntegerOverflow=on  InputSameDT=on
  Product : Product  Inputs=*/  SaturateOnIntegerOverflow=on  InputSameDT=on
  Switch : Switch  Threshold=1e-6  SaturateOnIntegerOverflow=on  InputSameDT=on
  Tm : Outport
  tag scope: w_ASM=global
  wires:
  w_Turb/1 -> 1800 rpm/1, Switch/1, Switch/2, [w_ASM]
  Constant3/1 -> Switch/3
  w_Wind/1 -> P(w_Wind,w_Turb)/1
  P(w_Wind,w_Turb)/1 -> Product/1
  Switch/1 -> Product/2
  Product/1 -> Gain/1
  Gain/1 -> Tm/1
  1800 rpm/1 -> P(w_Wind,w_Turb)/2

== system psbwindgen/Frequency Regulator/PD ==
  In : Inport  Port=1  LatchInput=off
  "0, 255" : Saturate  UpperLimit=255  LowerLimit=0
  Gain I : Gain  Gain=Kd  SaturateOnIntegerOverflow=on
  Gain P : Gain  Gain=Kp  SaturateOnIntegerOverflow=on
  Sum : Sum  SaturateOnIntegerOverflow=on  InputSameDT=on
  Transfer Fcn : TransferFcn  Numerator=[1 0]  Denominator=[1e-3 1]
  Out : Outport
  wires:
  Transfer Fcn/1 -> Sum/2
  "0, 255"/1 -> Out/1
  Gain I/1 -> Transfer Fcn/1
  In/1 -> Gain P/1, Gain I/1
  Gain P/1 -> Sum/1
  Sum/1 -> "0, 255"/1

== system psbwindgen/Frequency Regulator/Pulses Decoder ==
  Code : Inport  Port=1  LatchInput=off
  Constant : Constant  Value=pow2(0:-1:-(n-1))
  Constant6 : Constant  Value=2
  Math Function : Math  Operator=rem  SaturateOnIntegerOverflow=on
  Product : Product  SaturateOnIntegerOverflow=on  InputSameDT=on
  Rounding Function : Rounding
  Pulses : Outport
  wires:
  Math Function/1 -> Pulses/1
  Rounding Function/1 -> Math Function/1
  Constant6/1 -> Math Function/2
  Product/1 -> Rounding Function/1
  Code/1 -> Product/1
  Constant/1 -> Product/2

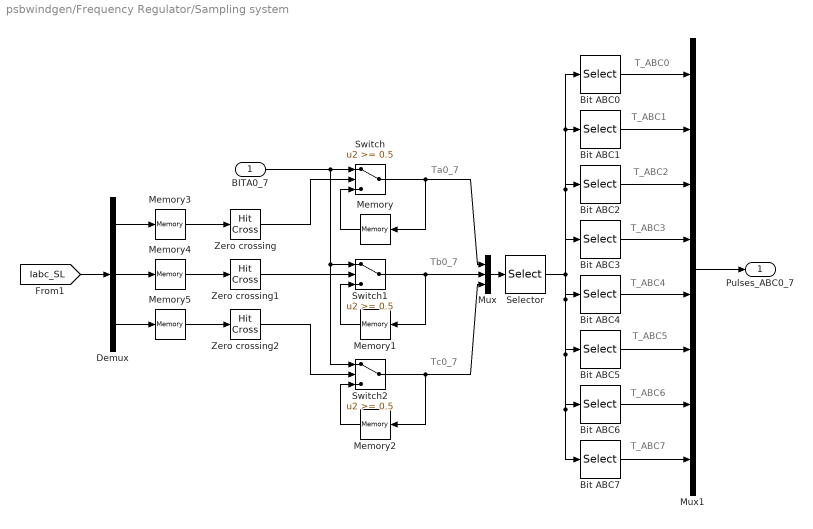
== system psbwindgen/Frequency Regulator/Sampling system ==
  note: T_ABC7
  note: T_ABC6
  note: T_ABC5
  note: T_ABC4
  note: T_ABC3
  note: T_ABC2
  note: T_ABC1
  note: T_ABC0
  note: Tc0_7
  note: Tb0_7
  note: Ta0_7
  BITA0_7 : Inport  Port=1  LatchInput=off
  " Bit ABC4" : Selector  Elements=[13 14 15]  InputPortWidth=24
  Bit ABC0 : Selector  Elements=[1 2 3]  InputPortWidth=24
  Bit ABC1 : Selector  Elements=[4 5 6]  InputPortWidth=24
  Bit ABC2 : Selector  Elements=[7 8 9]  InputPortWidth=24
  Bit ABC3 : Selector  Elements=[10 11 12]  InputPortWidth=24
  Bit ABC5 : Selector  Elements=[16 17 18]  InputPortWidth=24
  Bit ABC6 : Selector  Elements=[19 20 21]  InputPortWidth=24
  Bit ABC7 : Selector  Elements=[22 23 24]  InputPortWidth=24
  Demux : Demux  Outputs=3
  Memory : Memory  Orientation=left
  Memory1 : Memory  Orientation=left
  Memory2 : Memory  Orientation=left
  Memory3 : Memory
  Memory4 : Memory
  Memory5 : Memory
  Mux : Mux  Inputs=3
  Mux1 : Mux  Inputs=8
  Selector : Selector  Elements=[1 9 17 2 10 18 3 11 19 4 12 20 5 13 21 6 14 22 7 15 23 8 16 24]  InputPortWidth=24
  Switch : Switch  Threshold=0.5  SaturateOnIntegerOverflow=on  InputSameDT=on
  Switch1 : Switch  Threshold=0.5  SaturateOnIntegerOverflow=on  InputSameDT=on
  Switch2 : Switch  Threshold=0.5  SaturateOnIntegerOverflow=on  InputSameDT=on
  Zero crossing : HitCross
  Zero crossing1 : HitCross
  Zero crossing2 : HitCross
  Pulses_ABC0_7 : Outport
  wires:
  BITA0_7/1 -> Switch2/1, Switch1/1, Switch/1
  Memory5/1 -> Zero crossing2/1
  Memory4/1 -> Zero crossing1/1
  Memory3/1 -> Zero crossing/1
  Demux/3 -> Memory5/1
  Demux/2 -> Memory4/1
  Demux/1 -> Memory3/1
  Zero crossing2/1 -> Switch2/2
  Zero crossing1/1 -> Switch1/2
  Zero crossing/1 -> Switch/2
  [Iabc_SL] -> Demux/1
  Mux1/1 -> Pulses_ABC0_7/1
  Bit ABC7/1 -> Mux1/8
  Bit ABC6/1 -> Mux1/7
  Bit ABC5/1 -> Mux1/6
  " Bit ABC4"/1 -> Mux1/5
  Bit ABC3/1 -> Mux1/4
  Bit ABC2/1 -> Mux1/3
  Bit ABC1/1 -> Mux1/2
  Bit ABC0/1 -> Mux1/1
  Selector/1 -> Bit ABC7/1, Bit ABC6/1, Bit ABC5/1, " Bit ABC4"/1, Bit ABC3/1, Bit ABC2/1, Bit ABC0/1, Bit ABC1/1
  Mux/1 -> Selector/1
  Memory2/1 -> Switch2/3
  Switch2/1 -> Mux/3, Memory2/1
  Memory1/1 -> Switch1/3
  Switch1/1 -> Mux/2, Memory1/1
  Memory/1 -> Switch/3
  Switch/1 -> Mux/1, Memory/1

== system psbwindgen/Load/Ia ==
  Out1 : Outport
  wires:
  [tp575114] -> Out1/1

== system psbwindgen/Load/Ib ==
  Out1 : Outport
  wires:
  [tp575115] -> Out1/1

== system psbwindgen/Load/Ic ==
  Out1 : Outport
  wires:
  [tp575116] -> Out1/1

== system psbwindgen/Load/Vb ==
  Out1 : Outport
  wires:
  [tp575112] -> Out1/1

== system psbwindgen/Load/Vc ==
  Out1 : Outport
  wires:
  [tp575113] -> Out1/1

== system psbwindgen/SC/Ia ==
  Out1 : Outport
  wires:
  [tp575122] -> Out1/1

== system psbwindgen/SC/Ib ==
  Out1 : Outport
  wires:
  [tp575123] -> Out1/1

== system psbwindgen/SC/Ic ==
  Out1 : Outport
  wires:
  [tp575124] -> Out1/1

== system psbwindgen/SC/Vb ==
  Out1 : Outport
  wires:
  [tp575120] -> Out1/1

== system psbwindgen/SC/Vc ==
  Out1 : Outport
  wires:
  [tp575121] -> Out1/1

== system psbwindgen/SL/Ia ==
  Out1 : Outport
  wires:
  [tp575130] -> Out1/1

== system psbwindgen/SL/Ib ==
  Out1 : Outport
  wires:
  [tp575131] -> Out1/1

== system psbwindgen/SL/Ic ==
  Out1 : Outport
  wires:
  [tp575132] -> Out1/1

== system psbwindgen/SL/Vb ==
  Out1 : Outport
  wires:
  [tp575128] -> Out1/1

== system psbwindgen/SL/Vc ==
  Out1 : Outport
  wires:
  [tp575129] -> Out1/1

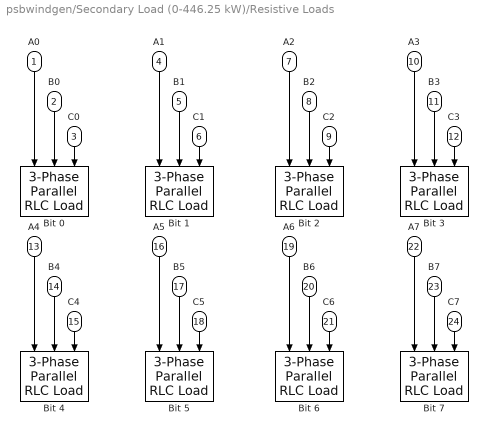
== system psbwindgen/Secondary Load (0-446.25 kW)/Resistive Loads ==
  A0 : Inport  Orientation=down  Port=1  LatchInput=off
  B0 : Inport  Orientation=down  Port=2  LatchInput=off
  C0 : Inport  Orientation=down  Port=3  LatchInput=off
  A1 : Inport  Orientation=down  Port=4  LatchInput=off
  B1 : Inport  Orientation=down  Port=5  LatchInput=off
  C1 : Inport  Orientation=down  Port=6  LatchInput=off
  A2 : Inport  Orientation=down  Port=7  LatchInput=off
  B2 : Inport  Orientation=down  Port=8  LatchInput=off
  C2 : Inport  Orientation=down  Port=9  LatchInput=off
  A3 : Inport  Orientation=down  Port=10  LatchInput=off
  B3 : Inport  Orientation=down  Port=11  LatchInput=off
  C3 : Inport  Orientation=down  Port=12  LatchInput=off
  A4 : Inport  Orientation=down  Port=13  LatchInput=off
  B4 : Inport  Orientation=down  Port=14  LatchInput=off
  C4 : Inport  Orientation=down  Port=15  LatchInput=off
  A5 : Inport  Orientation=down  Port=16  LatchInput=off
  B5 : Inport  Orientation=down  Port=17  LatchInput=off
  C5 : Inport  Orientation=down  Port=18  LatchInput=off
  A6 : Inport  Orientation=down  Port=19  LatchInput=off
  B6 : Inport  Orientation=down  Port=20  LatchInput=off
  C6 : Inport  Orientation=down  Port=21  LatchInput=off
  A7 : Inport  Orientation=down  Port=22  LatchInput=off
  B7 : Inport  Orientation=down  Port=23  LatchInput=off
  C7 : Inport  Orientation=down  Port=24  LatchInput=off
  Bit 0 : powerlib2/Elements/3-Phase Parallel RLC Load  Orientation=down  Vpp=Vphase_phase_lissage  fn=Freq  P3=P_lissage_min  QL3=0  QC3=0
  Bit 1 : powerlib2/Elements/3-Phase Parallel RLC Load  Orientation=down  Vpp=Vphase_phase_lissage  fn=Freq  P3=2*P_lissage_min  QL3=0  QC3=0
  Bit 2 : powerlib2/Elements/3-Phase Parallel RLC Load  Orientation=down  Vpp=Vphase_phase_lissage  fn=Freq  P3=2^2*P_lissage_min  QL3=0  QC3=0
  Bit 3 : powerlib2/Elements/3-Phase Parallel RLC Load  Orientation=down  Vpp=Vphase_phase_lissage  fn=Freq  P3=2^3*P_lissage_min  QL3=0  QC3=0
  Bit 4 : powerlib2/Elements/3-Phase Parallel RLC Load  Orientation=down  Vpp=Vphase_phase_lissage  fn=Freq  P3=2^4*P_lissage_min  QL3=0  QC3=0
  Bit 5 : powerlib2/Elements/3-Phase Parallel RLC Load  Orientation=down  Vpp=Vphase_phase_lissage  fn=Freq  P3=2^5*P_lissage_min  QL3=0  QC3=0
  Bit 6 : powerlib2/Elements/3-Phase Parallel RLC Load  Orientation=down  Vpp=Vphase_phase_lissage  fn=Freq  P3=2^6*P_lissage_min  QL3=0  QC3=0
  Bit 7 : powerlib2/Elements/3-Phase Parallel RLC Load  Orientation=down  Vpp=Vphase_phase_lissage  fn=Freq  P3=2^7*P_lissage_min  QL3=0  QC3=0
  wires:
  C7/1 -> Bit 7/3
  B7/1 -> Bit 7/2
  A7/1 -> Bit 7/1
  C6/1 -> Bit 6/3
  B6/1 -> Bit 6/2
  A6/1 -> Bit 6/1
  C5/1 -> Bit 5/3
  B5/1 -> Bit 5/2
  A5/1 -> Bit 5/1
  C4/1 -> Bit 4/3
  B4/1 -> Bit 4/2
  A4/1 -> Bit 4/1
  C3/1 -> Bit 3/3
  B3/1 -> Bit 3/2
  A3/1 -> Bit 3/1
  C2/1 -> Bit 2/3
  B2/1 -> Bit 2/2
  A2/1 -> Bit 2/1
  C1/1 -> Bit 1/3
  B1/1 -> Bit 1/2
  A1/1 -> Bit 1/1
  C0/1 -> Bit 0/3
  B0/1 -> Bit 0/2
  A0/1 -> Bit 0/1
